simulink model "AutosarStructrueTemplete"  (R2023b)
settings: Solver=FixedStepDiscrete  StartTime=0.0  StopTime=10.0  FixedStep=0.02  RelTol=1e-3  EnableMultiTasking=on
undefined symbols (not defined in the file or in its folder): D1, P
libraries: autosarlibdem x1, autosarlibnvm x1
settings Model: DataDictionary=autosar.sldd  Creator=admin  LastModifiedBy=admin
settings SolverCC: AlgebraicLoopSolver=TrustRegion  AutoInsertRateTranBlk=on  InsertRTBMode=Never (minimum delay)  MaxZcPerStep=1
settings OptimizationCC: DefaultParameterBehavior=Inlined  EnhancedBackFolding=on  PassReuseOutputArgsAs=Individual arguments  ZeroExternalMemoryAtStartup=off  ZeroInternalMemoryAtStartup=off  OptimizeBlockOrder=speed  DifferentSizesBufferReuse=on  OptimizationCustomize=off  EfficientTunableParamExpr=on
settings DebuggingCC: MultiTaskDSMMsg=none  MultiTaskRateTransMsg=warning  ParameterTunabilityLossMsg=error  UnconnectedLineMsg=warning
settings ModelReferenceCC: EnableRefExpFcnMdlSchedulingChecks=on
settings SFSimCC: MATLABDynamicMemAlloc=off
settings RTWCC: Description=AUTOSAR  SystemTargetFile=autosar.tlc  GenCodeOnly=on  TemplateMakefile=ert_default_tmf  IncludeHyperlinkInReport=on  DataTypeReplacement=CDataTypesFixedWidth  DLArmComputeVersion=19.05
settings CodeAppCC: ForceParamTrailComments=on  IgnoreCustomStorageClasses=off  OperatorAnnotations=on  SimulinkDataObjDesc=on  SFDataObjDesc=on  InsertBlockDesc=on
settings STFCustomTargetCC: MultiwordLength=256  ParMdlRefBuildCompliant=on  CompOptLevelCompliant=on  IncludeMdlTerminateFcn=off  CombineOutputUpdateFcns=on  SuppressErrorStatus=on  ERTCustomFileBanners=on  SupportNonFinite=off  SupportComplex=off  SupportContinuousTime=off  SupportNonInlinedSFcns=off  RemoveResetFunc=on  MATLABClassNameForMDSCustomization=Simulink.SoftwareTarget.ERTCustomization  AutosarCompliant=on  UseToolchainInfoCompliant=on  LookupTableObjectStructAxisOrder=2,1,3,4,...  LUTObjectStructOrderEvenSpacing=Size,Table,Breakpoints  SystemTargetFile=autosar.tlc
settings ERTTargetCC: TargetLangStandard=C99 (ISO)  ConcurrentExecutionCompliant=off  IncludeMdlTerminateFcn=off  SuppressErrorStatus=on  SupportNonFinite=off  SupportComplex=off  ModelStepFunctionPrototypeControlCompliant=off  CPPClassGenCompliant=off  AutosarCompliant=on  LookupTableObjectStructAxisOrder=2,1,3,4,...  LUTObjectStructOrderEvenSpacing=Size,Table,Breakpoints  InlinedParameterPlacement=NonHierarchical  ERTCustomFileTemplate=example_file_process.tlc

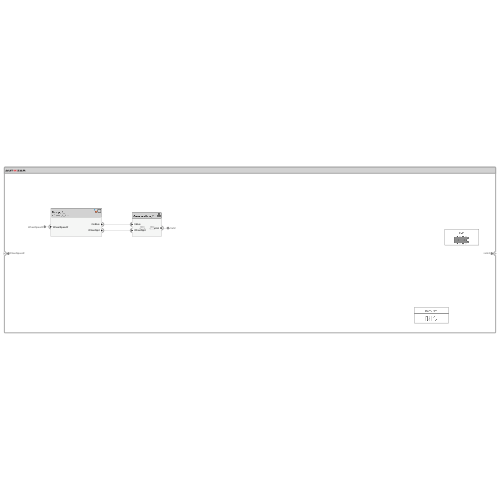
[thumbnail: Simulink's stored preview of the top-level diagram]
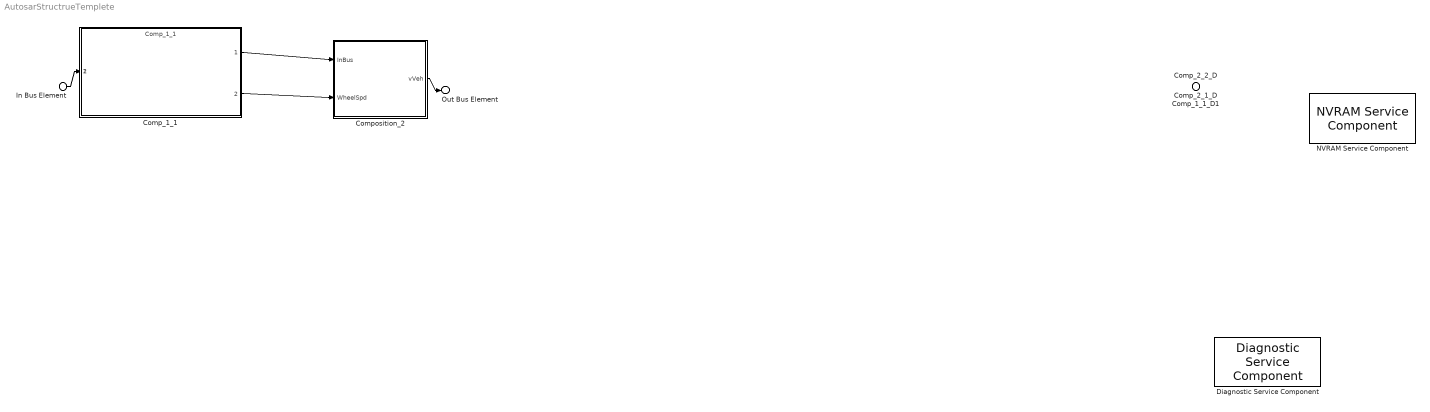
== system AutosarStructrueTemplete ==
  In Bus Element : Inport  PortName=WheelSpeedF
  Comp_2_1_D : Inport  Port=2  OutputFunctionCall=on
  Comp_2_2_D : Inport  Port=3  OutputFunctionCall=on
  Comp_1_1_D1 : Inport  Port=4  OutputFunctionCall=on
  Comp_1_1 : ModelReference  ModelNameDialog=Comp_1_1  SimulationMode=Normal  ScheduleRates=on  CachedPortDiscreteRates=[1]  ModelEventPortInfo=P:D1[1][0][0]  CodeInterface=Top model  ModelReferenceVersion=1.21
      settings: PortSchema="{\"entries\":[{\"content\":{\"headerSize\":38,\"margin\":15,\"minimumSpacing\":25,\"sides\":[{\"content\":{\"connectorIds\":[\"In1\"]},\"type\":\"ConnectorPlacement.EquallySpacedRectSide\",\"uuid\":\"2c931de4-069c-498e-9ead-a157c6c26d81\"},{\"content\":{\"connectorIds\":[\"Out1\",\"Out2\"],\"side\":\"RIGHT\"},\"type\":\"ConnectorPlacement.EquallySpacedRectSide\",\"uuid\":\"f36afbb2-17c7-4f32-ab7c-6686c2a85676\"},{\"content\":{\"side\":\"TOP\"},\"type\":\"ConnectorPlacement.EquallySpacedRectSide\",\"uuid\":\"6cbfe0c2-7bd7-405e-91f9-cdacb3fa9c4a\"},{\"content\":{\"connectorIds\":[\"In2\"],\"side\":\"HIDDEN\"},\"type\":\"ConnectorPlacement.EquallySpacedRectSide\",\"uuid\":\"d8bdbca5-46b4-43ac-b2d4-ed5eebd53d91\"}]},\"type\":\"ConnectorPlacement.EquallySpacedConnector\",\"uuid\":\"9e22a0e1-d5b0-4cbb-b83e-b8bd2254246c\"}],\"packageUris\":[\"http://schema.mathworks.com/mf0/Connector/R2020b\"],\"version\":\"1.0\"}"
  Composition_2 : Subsystem
      settings: PortSchema="{\"entries\":[{\"content\":{\"headerSize\":26,\"margin\":15,\"minimumSpacing\":25,\"sides\":[{\"content\":{\"connectorIds\":[\"In1\",\"In2\"]},\"type\":\"ConnectorPlacement.EquallySpacedRectSide\",\"uuid\":\"f42b55a5-1b3b-4a57-aff4-096db973c6eb\"},{\"content\":{\"connectorIds\":[\"Out1\"],\"side\":\"RIGHT\"},\"type\":\"ConnectorPlacement.EquallySpacedRectSide\",\"uuid\":\"bfed65a7-8979-4e26-b411-2100b7eb35e8\"},{\"content\":{\"side\":\"TOP\"},\"type\":\"ConnectorPlacement.EquallySpacedRectSide\",\"uuid\":\"0a83ab61-8db2-4d3b-88b8-f344af21d74d\"}]},\"type\":\"ConnectorPlacement.EquallySpacedConnector\",\"uuid\":\"ed527a4b-e081-4d85-8320-14a54c3a3837\"}],\"packageUris\":[\"http://schema.mathworks.com/mf0/Connector/R2020b\"],\"version\":\"1.0\"}"
  Diagnostic Service Component : autosarlibdem/Diagnostic Service Component  ClientPortNames={}  ClientPortPortDefinedArguments={}  MaxEventId=10  MaxFID=10  DemDebounceCounterIncrementStepSize=1  DemDebounceCounterDecrementStepSize=1  DemDebounceCounterFailedThreshold=2  DemDebounceCounterPassedThreshold=-1  InhibitionMatrix=zeros(11,'uint8')  EnableConditionIndexes=zeros(257,'uint8')  StorageConditionIndexes=zeros(257,'uint8')
  NVRAM Service Component : autosarlibnvm/NVRAM Service Component  ClientPortNames={}  ClientPortPortDefinedArguments={}  MaxBlockId=10  NvInitValues={'0'}
  Out Bus Element : Outport  PortName=vVehF
  wires:
  In Bus Element/1 -> Comp_1_1/1
  Composition_2/1(vVeh) -> Out Bus Element/1
  Comp_1_1/2 -> Composition_2/2(WheelSpd)
  Comp_1_1/1 -> Composition_2/1(InBus)

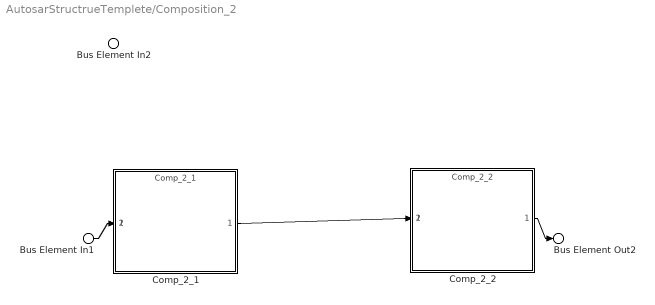
== system AutosarStructrueTemplete/Composition_2 ==
  Bus Element In2 : Inport  PortName=InBus
  Bus Element In1 : Inport  Port=2  PortName=WheelSpd
  Comp_2_1 : ModelReference  ModelNameDialog=Comp_2_1  SimulationMode=Normal  ScheduleRates=on  CachedPortDiscreteRates=[-1]  ModelEventPortInfo=P:D1[-1][0][0]  CodeInterface=Top model  ModelReferenceVersion=1.13
      settings: PortSchema="{\"entries\":[{\"content\":{\"headerSize\":38,\"margin\":15,\"minimumSpacing\":25,\"sides\":[{\"content\":{\"connectorIds\":[\"In1\"]},\"type\":\"ConnectorPlacement.EquallySpacedRectSide\",\"uuid\":\"f42b55a5-1b3b-4a57-aff4-096db973c6eb\"},{\"content\":{\"connectorIds\":[\"Out1\"],\"side\":\"RIGHT\"},\"type\":\"ConnectorPlacement.EquallySpacedRectSide\",\"uuid\":\"bfed65a7-8979-4e26-b411-2100b7eb35e8\"},{\"content\":{\"side\":\"TOP\"},\"type\":\"ConnectorPlacement.EquallySpacedRectSide\",\"uuid\":\"0a83ab61-8db2-4d3b-88b8-f344af21d74d\"},{\"content\":{\"connectorIds\":[\"In2\"],\"side\":\"HIDDEN\"},\"type\":\"ConnectorPlacement.EquallySpacedRectSide\",\"uuid\":\"62fa3b87-108a-43dd-a1ea-25a2cb8a7350\"}]},\"type\":\"ConnectorPlacement.EquallySpacedConnector\",\"uuid\":\"ed527a4b-e081-4d85-8320-14a54c3a3837\"}],\"packageUris\":[\"http://schema.mathworks.com/mf0/Connector/R2020b\"],\"version\":\"1.0\"}"
  Comp_2_2 : ModelReference  ModelNameDialog=Comp_2_2  SimulationMode=Normal  ScheduleRates=on  CachedPortDiscreteRates=[-1]  ModelEventPortInfo=P:D1[-1][0][0]  CodeInterface=Top model  ModelReferenceVersion=1.11
      settings: PortSchema="{\"entries\":[{\"content\":{\"headerSize\":38,\"margin\":15,\"minimumSpacing\":25,\"sides\":[{\"content\":{\"connectorIds\":[\"In1\"]},\"type\":\"ConnectorPlacement.EquallySpacedRectSide\",\"uuid\":\"f42b55a5-1b3b-4a57-aff4-096db973c6eb\"},{\"content\":{\"connectorIds\":[\"Out1\"],\"side\":\"RIGHT\"},\"type\":\"ConnectorPlacement.EquallySpacedRectSide\",\"uuid\":\"bfed65a7-8979-4e26-b411-2100b7eb35e8\"},{\"content\":{\"side\":\"TOP\"},\"type\":\"ConnectorPlacement.EquallySpacedRectSide\",\"uuid\":\"0a83ab61-8db2-4d3b-88b8-f344af21d74d\"},{\"content\":{\"connectorIds\":[\"In2\"],\"side\":\"HIDDEN\"},\"type\":\"ConnectorPlacement.EquallySpacedRectSide\",\"uuid\":\"5227266b-9603-4589-a177-8eecd2f40188\"}]},\"type\":\"ConnectorPlacement.EquallySpacedConnector\",\"uuid\":\"ed527a4b-e081-4d85-8320-14a54c3a3837\"}],\"packageUris\":[\"http://schema.mathworks.com/mf0/Connector/R2020b\"],\"version\":\"1.0\"}"
  Bus Element Out2 : Outport  PortName=vVeh
  wires:
  Bus Element In1/1 -> Comp_2_1/1
  Comp_2_1/1 -> Comp_2_2/1
  Comp_2_2/1 -> Bus Element Out2/1
